simulink library "rotationFromTangentToBody"  (R2020a)
settings: Solver=VariableStepAuto  StartTime=0.0  StopTime=10.0  RelTol=1e-3
libraries: rotationAboutX x1, rotationAboutY x1, rotationAboutZ x1
settings Model: Creator=Ayaz  LastModifiedBy=Ayaz

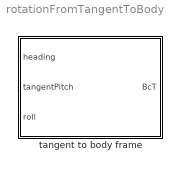
== system rotationFromTangentToBody ==
  tangent to body frame : Subsystem

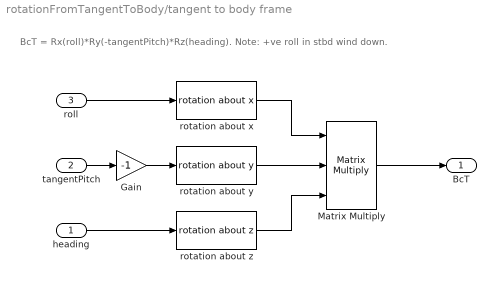
== system rotationFromTangentToBody/tangent to body frame ==
  note: BcT = Rx(roll)*Ry(-tangentPitch)*Rz(heading). Note: +ve roll in stbd wind down.
  heading : Inport
  tangentPitch : Inport  Port=2
  roll : Inport  Port=3
  Gain : Gain  Gain=-1
  Matrix Multiply : Product  Inputs=3  Multiplication=Matrix(*)
  rotation about x : rotationAboutX/rotation about x  SystemSampleTime=-1  Latency=0  AutoFrameSizeCalculation=off
  rotation about y : rotationAboutY/rotation about y  SystemSampleTime=-1  Latency=0  AutoFrameSizeCalculation=off
  rotation about z : rotationAboutZ/rotation about z  SystemSampleTime=-1  Latency=0  AutoFrameSizeCalculation=off
  BcT : Outport
  wires:
  heading/1 -> rotation about z/1
  tangentPitch/1 -> Gain/1
  roll/1 -> rotation about x/1
  rotation about y/1 -> Matrix Multiply/2
  Matrix Multiply/1 -> BcT/1
  rotation about x/1 -> Matrix Multiply/1
  rotation about z/1 -> Matrix Multiply/3
  Gain/1 -> rotation about y/1
